simulink model "orc2_GyroSimulation"  (R2014b)
settings: Solver=ode3  StartTime=0.0  StopTime=70.000424  FixedStep=ts  RelTol=1e-6
InitFcn:
  | InitGyro
undefined symbols (not defined in the file or in its folder): Dr, Du, select_controller, sigbuilder_block
undefined symbols (not defined in the file): q1dot_0, q2_0, q3_0, sys
libraries: simulink_extras x5, cstblocks x4, simulink x1
settings Model: Creator=jt  LastModifiedBy=sv
settings OptimizationCC: UseDivisionForNetSlopeComputation=off  SimCompilerOptimization=off
settings DebuggingCC: UnderspecifiedInitializationDetection=Classic  MergeDetectMultiDrivingBlocksExec=none  FrameProcessingCompatibilityMsg=error  StateNameClashWarn=warning
settings RTWCC: RTWCompilerOptimization=off

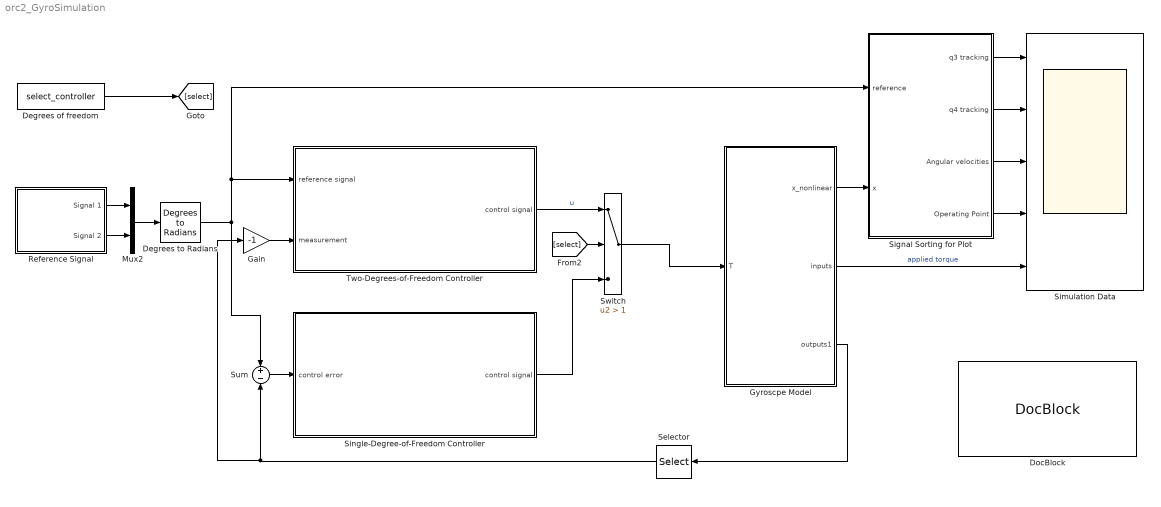
== system orc2_GyroSimulation ==
  Degrees of freedom : Constant  Value=select_controller
  Degrees to Radians : simulink_extras/Transformations/Degrees to Radians
  DocBlock : simulink/Model-Wide Utilities/DocBlock  DocumentType=Text
      content=|
      | % #########################################################################
      | % TUHH :: Institute for Control Systems :: Control Lab
      | % #########################################################################
      | % Experiment ORC2: Robust Control of a Gyroscope
      | %
      | % Copyright Herbert Werner and Hamburg University of Technology, 2014
      | % #########################################################################
      | % This is the experiment interface, tested with Matlab2014b 64bit
      | %
      | % Make sure you run the file orc2_experiment to set necessary parameters.
      | % Further, the following variables need to be in the workspace to run the
      | % experiment:
      | %  - K1 [ss]        : single-degree-of-freedom controller
      | %  - K2 [ss]        : two-degrees-of-freedom controller
      | %  - Du [double]    : plant input scaling
      | %  - Dr [double]    : plant output scaling
      |
      | %----------------------------
      | % v.0.8b1 - 21-01-2015
      | % by Julian Theis
      | %----------------------------
      | % Last modified on 21-01-2015
      | % by Julian Theis
      | % ---------------------------
  Gain : Gain  Gain=-1
  Gyroscpe Model : Subsystem
  Mux2 : Mux  Inputs=2
  Reference Signal : Subsystem  Tag=STV Subsys  LoadFcn=sigbuilder_block('load');  StartFcn=sigbuilder_block('start');  StopFcn=sigbuilder_block('stop');  ClipboardFcn=sigbuilder_block('clipboard');  mask(Sigbuilder block){}
      mask help: Sigbuilder GUI
      mask init:
      | if ~strcmp(get_param(bdroot(gcbh),'SimulationStatus'),'stopped') tuvar = sigbuilder_block('maskInit'); end
      settings: CopyFcn=sigbuilder_block('copy');  DeleteFcn=sigbuilder_block('delete');  ModelCloseFcn=sigbuilder_block('modelClose');  PreSaveFcn=sigbuilder_block('preSave');  PauseFcn=sigbuilder_block('pause')  ContinueFcn=sigbuilder_block('continue')  NameChangeFcn=sigbuilder_block('namechange');  OpenFcn=sigbuilder_block('open',[6 0 1428 718.5 ]);  CloseFcn=sigbuilder_block('close');
      mask Display: plot(0,0,100,100,[10,10,40,40,10],[80,20,20,80,80],[40,10],[50,50], [40,27,10],[65,72,56],[40,25,25,10],[28,28,43,43]);
  Selector : Selector  InputPortWidth=4  Indices=[1 2]
  Signal Sorting for Plot : Subsystem
  Simulation Data : Scope  NumInputPorts=5
      settings: TickLabels=on  TimeRange=70.000424  YMin=-10~-100~-2~-20~-2  YMax=10~100~2~60~2  SaveName=simdata
  Single-Degree-of-Freedom Controller : Subsystem
  Sum : Sum  Inputs=+|-
  Switch : Switch  Criteria=u2 > Threshold  Threshold=1
  Two-Degrees-of-Freedom Controller : Subsystem
  wires:
  Switch/1 -> Gyroscpe Model/1(T)
  Two-Degrees-of-Freedom Controller/1(control signal) -> Switch/1  "u"
  Gyroscpe Model/2(inputs) -> Simulation Data/5  "applied torque"
  Gyroscpe Model/1(x_nonlinear) -> Signal Sorting for Plot/2(x)
  Gyroscpe Model/3(outputs1) -> Selector/1
  Signal Sorting for Plot/1(q3 tracking) -> Simulation Data/1
  Signal Sorting for Plot/2(q4 tracking) -> Simulation Data/2
  Signal Sorting for Plot/3(Angular velocities) -> Simulation Data/3
  Signal Sorting for Plot/4(Operating Point) -> Simulation Data/4
  [select] -> Switch/2
  Degrees of freedom/1 -> [select]
  Single-Degree-of-Freedom Controller/1(control signal) -> Switch/3
  Sum/1 -> Single-Degree-of-Freedom Controller/1(control error)
  Gain/1 -> Two-Degrees-of-Freedom Controller/2(measurement)
  Degrees to Radians/1 -> Sum/1, Two-Degrees-of-Freedom Controller/1(reference signal), Signal Sorting for Plot/1(reference)
  Mux2/1 -> Degrees to Radians/1
  Reference Signal/1(Signal 1) -> Mux2/1
  Reference Signal/2(Signal 2) -> Mux2/2
  Selector/1 -> Gain/1, Sum/2

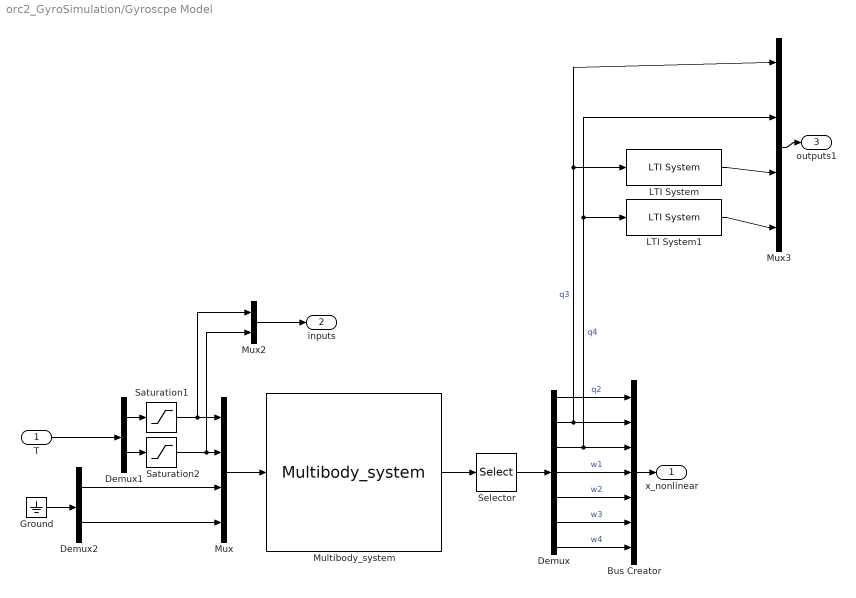
== system orc2_GyroSimulation/Gyroscpe Model ==
  T : Inport
  Bus Creator : BusCreator  Inputs=7
  Demux : Demux  Outputs=7
  Demux1 : Demux  Outputs=2
  Demux2 : Demux  Outputs=2
  Ground : Ground
  LTI System : cstblocks/LTI System  sys=diff_filter  IC=[]
  LTI System1 : cstblocks/LTI System  sys=diff_filter  IC=[]
  Multibody_system : S-Function  FunctionName=Multibody_system  Parameters=paraStruct, initY, initDy  EnableBusSupport=off  mask(Neweul-M2 nonlinear model){paraStruct=sys.parameters.data, initY=[0 q2_0 q3_0 0]';, initDy=[q1dot_0 0 0 0]';}
      mask prompts: paraStruct "Neweul-M2 Parameter Structure"; initY "Initial coordinates"; initDy "Initial velocities"
      mask help:
      | State-state representation of a multibody system
      | created with Neueul-MÂ².
      |
      | In order to run a simulation in Simulink you have to provide
      | the following input parameters:
      |   * Neweul-M2 Parameter Structure (sys.parameters.data)
      |     ... Structure containing all user-defined parameters
      |   * Initial coordinates (zeros(sys.counters.genCoord,1))
      |     ... Initial values for the generalized coordinates
      |   * Initial velocities (zeros(sys.dof,1))
      |     ... Initial values for the generalized velocities
      |
      | Neweul-MÂ²
      | Multibody systems based on symbolic Newton-Euler-Equations
      | Copyright (c) ITM University of Stuttgart, www.itm.uni-stuttgart.de
      mask Display:
      | port_label('output',1,'states [8x1]');
      | port_label('input',1,'control [4x1]');
  Mux : Mux
  Mux2 : Mux  Inputs=2
  Mux3 : Mux
  Saturation1 : Saturate  UpperLimit=0.666  LowerLimit=-0.666
  Saturation2 : Saturate  UpperLimit=2.44  LowerLimit=-2.44
  Selector : Selector  Indices=2:8
  x_nonlinear : Outport
  inputs : Outport  Port=2
  outputs1 : Outport  Port=3
  wires:
  Multibody_system/1 -> Selector/1
  Demux/6 -> Bus Creator/6  "w3"
  Demux/1 -> Bus Creator/1  "q2"
  Demux/7 -> Bus Creator/7  "w4"
  Selector/1 -> Demux/1
  Bus Creator/1 -> x_nonlinear/1
  Mux/1 -> Multibody_system/1
  Demux2/2 -> Mux/4
  Demux2/1 -> Mux/3
  Demux1/2 -> Saturation2/1
  Demux/5 -> Bus Creator/5  "w2"
  Demux/4 -> Bus Creator/4  "w1"
  Mux2/1 -> inputs/1
  Saturation2/1 -> Mux2/2, Mux/2
  Saturation1/1 -> Mux2/1, Mux/1
  Demux1/1 -> Saturation1/1
  T/1 -> Demux1/1
  Ground/1 -> Demux2/1
  Demux/3 -> Bus Creator/3, LTI System1/1, Mux3/2  "q4"
  Demux/2 -> Bus Creator/2, Mux3/1, LTI System/1  "q3"
  Mux3/1 -> outputs1/1
  LTI System/1 -> Mux3/3
  LTI System1/1 -> Mux3/4

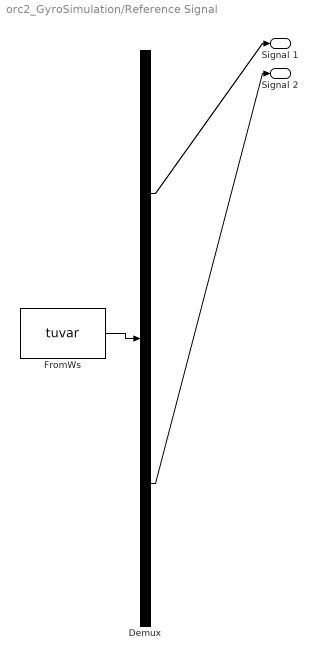
== system orc2_GyroSimulation/Reference Signal ==
  Demux : Demux  Tag=STV Demux  Outputs=2
  FromWs : FromWorkspace  Tag=STV FromWs  VariableName=tuvar  SampleTime=0
      SigBuilderData=|
      | common.afterFinalStr = 'Extrapolate'
      | common.sampleTime = 0
      | dataSet.timeRange = [0 70]
      | dataSet.name = 'Group 1'
      | sbobj.Groups.Name = 'Group 1'
      | sbobj.Groups.Signals(1).Name = 'Signal 1'
      | sbobj.Groups.Signals(1).XData = [0 22 22 28 28 34 34 40 40 46 46 52 52 58 58 64 64 70]
      | sbobj.Groups.Signals(1).YData = [0 0 -5 -5 0 0 5 5 0 0 -5 -5 0 0 5 5 0 0]
      | sbobj.Groups.Signals(2).Name = 'Signal 2'
      | sbobj.Groups.Signals(2).XData = [0 25 25 37 37 49 49 61 61 70]
      | sbobj.Groups.Signals(2).YData = [0 0 -40 -40 0 -0.2 40 40 -0.2 -0.2]
      | sbobj.Groups.TimeRange = [0 70]
  Signal 1 : Outport  Tag=STV Outport
  Signal 2 : Outport  Tag=STV Outport  Port=2
  wires:
  FromWs/1 -> Demux/1
  Demux/1 -> Signal 1/1
  Demux/2 -> Signal 2/1

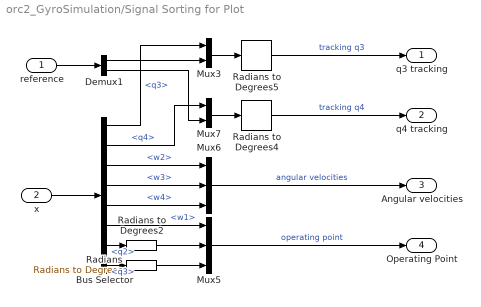
== system orc2_GyroSimulation/Signal Sorting for Plot ==
  reference : Inport
  x : Inport  Port=2
  Bus Selector : BusSelector  OutputSignals=q3,q4,w2,w3,w4,w1,q2,q3
  Demux1 : Demux  Outputs=2
  Mux3 : Mux  Inputs=2
  Mux5 : Mux  Inputs=3
  Mux6 : Mux  Inputs=3
  Mux7 : Mux  Inputs=2
  "Radians " : simulink_extras/Transformations/Radians to Degrees
  Radians to Degrees2 : simulink_extras/Transformations/Radians to Degrees
  Radians to Degrees4 : simulink_extras/Transformations/Radians to Degrees
  Radians to Degrees5 : simulink_extras/Transformations/Radians to Degrees
  q3 tracking : Outport
  q4 tracking : Outport  Port=2
  Angular velocities : Outport  Port=3
  Operating Point : Outport  Port=4
  wires:
  Bus Selector/3 -> Mux6/1  "<w2>"
  Bus Selector/2 -> Mux7/1  "<q4>"
  Radians to Degrees4/1 -> q4 tracking/1  "tracking q4"
  Mux3/1 -> Radians to Degrees5/1
  Radians to Degrees5/1 -> q3 tracking/1  "tracking q3"
  Mux7/1 -> Radians to Degrees4/1
  Demux1/1 -> Mux3/2
  Demux1/2 -> Mux7/2
  Bus Selector/1 -> Mux3/1  "<q3>"
  Mux6/1 -> Angular velocities/1  "angular velocities"
  Bus Selector/5 -> Mux6/3  "<w4>"
  Bus Selector/4 -> Mux6/2  "<w3>"
  Mux5/1 -> Operating Point/1  "operating point"
  Bus Selector/6 -> Mux5/1  "<w1>"
  Bus Selector/7 -> Radians to Degrees2/1  "<q2>"
  Bus Selector/8 -> "Radians "/1  "<q3>"
  "Radians "/1 -> Mux5/3
  Radians to Degrees2/1 -> Mux5/2
  reference/1 -> Demux1/1
  x/1 -> Bus Selector/1

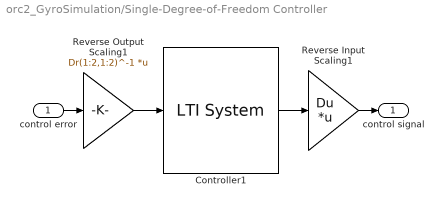
== system orc2_GyroSimulation/Single-Degree-of-Freedom Controller ==
  control error : Inport
  Controller1 : cstblocks/LTI System  sys=K1  IC=[]
  Reverse Input Scaling1 : Gain  Gain=Du  Multiplication=Matrix(K*u)
  Reverse Output Scaling1 : Gain  Gain=Dr(1:2,1:2)^-1  Multiplication=Matrix(K*u)
  control signal : Outport
  wires:
  control error/1 -> Reverse Output Scaling1/1
  Reverse Input Scaling1/1 -> control signal/1
  Controller1/1 -> Reverse Input Scaling1/1
  Reverse Output Scaling1/1 -> Controller1/1

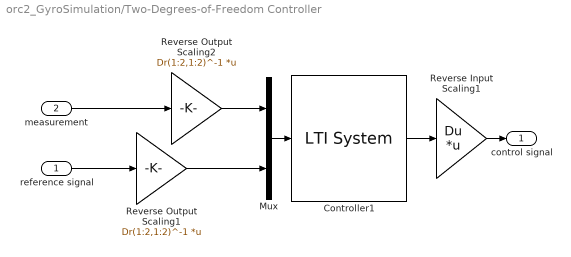
== system orc2_GyroSimulation/Two-Degrees-of-Freedom Controller ==
  reference signal : Inport
  measurement : Inport  Port=2
  Controller1 : cstblocks/LTI System  sys=K2  IC=[]
  Mux : Mux  Inputs=2
  Reverse Input Scaling1 : Gain  Gain=Du  Multiplication=Matrix(K*u)
  Reverse Output Scaling1 : Gain  Gain=Dr(1:2,1:2)^-1  Multiplication=Matrix(K*u)
  Reverse Output Scaling2 : Gain  Gain=Dr(1:2,1:2)^-1  Multiplication=Matrix(K*u)
  control signal : Outport
  wires:
  reference signal/1 -> Reverse Output Scaling1/1
  Reverse Input Scaling1/1 -> control signal/1
  Controller1/1 -> Reverse Input Scaling1/1
  Mux/1 -> Controller1/1
  measurement/1 -> Reverse Output Scaling2/1
  Reverse Output Scaling2/1 -> Mux/1
  Reverse Output Scaling1/1 -> Mux/2
